simulink model "normalization_tut"  (Simulink 5.0)
settings: Solver=FixedStepDiscrete  StartTime=0.0  StopTime=5  RelTol=1e-3
libraries: dspsigattribs x1, dspmathops x1, dspsrcs4 x1
settings Model: Creator=ckamachi  LastModifiedBy=ckamachi  ExtModeTrigMode=oneshot  ExtModeArmWhenConnect=off  LimitDataPoints=off  BlockReductionOpt=off  BooleanDataType=off

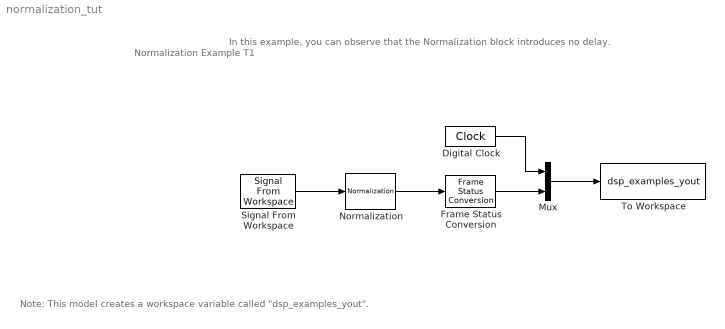
== system normalization_tut ==
  note: Normalization Example T1
  note: In this example, you can observe that the Normalization block
      | introduces no delay.
  note: Note: This model creates a workspace variable called "dsp_examples_yout".
  Digital Clock : DigitalClock
  Frame Status Conversion : dspsigattribs/Frame Status Conversion  growRefPort=off  outframe=Sample-based
  Mux : Mux  Inputs=2
  Normalization : dspmathops/Normalization  NormType=Squared 2-norm  Bias=1e-10
  Signal From Workspace : dspsrcs4/Signal From Workspace  X=1:100  Ts=1/4  nsamps=4  OutputAfterFinalValue=Setting to zero
  To Workspace : ToWorkspace  VariableName=dsp_examples_yout  SampleTime=-1  SaveFormat=Array
  wires:
  Normalization/1 -> Frame Status Conversion/1
  Signal From Workspace/1 -> Normalization/1
  Digital Clock/1 -> Mux/1
  Frame Status Conversion/1 -> Mux/2
  Mux/1 -> To Workspace/1
